simulink model "Modelo_lineal_5GDL_2022"  (R2021b)
settings: Solver=VariableStepAuto  StartTime=0.0  StopTime=0.1  MaxStep=1e-5  RelTol=1e-6
values from neighbouring files (symbols this model uses):
  g = 9.81    [main.m]
undefined symbols (not defined in the file or in its folder): A_EMS, A_HEMS, AG0, B_EMS, B_HEMS, beta, C_EMS, C_HEMS, D_EMS, D_HEMS, dTSensor, filterConstant, I_front, I_rear, initial_conds, noiseSensor, pod, ROTX_0, ROTY_0, ROTZ_0, y_ini, z_0, z_ini
libraries: shared6dof x1
(part 1 of 2)
settings Model: Creator=emate  LastModifiedBy=emate

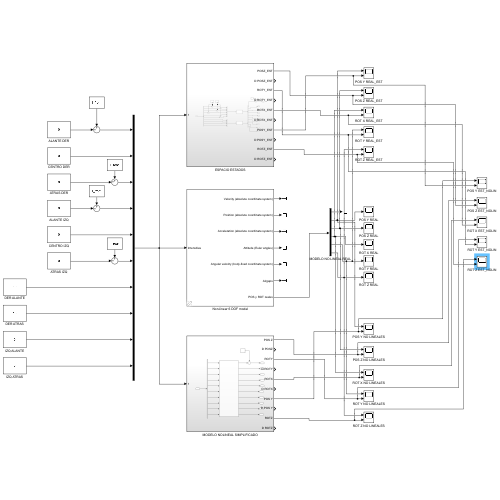
[thumbnail: Simulink's stored preview of the top-level diagram]
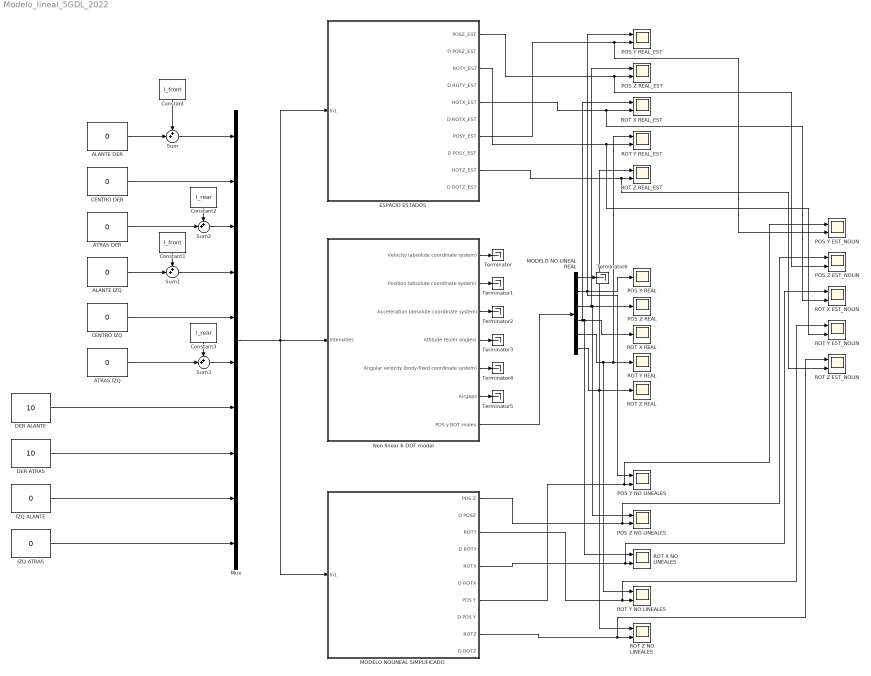
== system Modelo_lineal_5GDL_2022 ==
  ALANTE DER : Constant  Value=0
  ALANTE IZQ : Constant  Value=0
  ATRAS DER : Constant  Value=0
  ATRAS IZQ : Constant  Value=0
  CENTRO DER : Constant  Value=0
  CENTRO IZQ : Constant  Value=0
  Constant : Constant  Value=I_front
  Constant1 : Constant  Value=I_front
  Constant2 : Constant  Value=I_rear
  Constant3 : Constant  Value=I_rear
  DER ALANTE : Constant  Value=10
  DER ATRAS : Constant  Value=10
  ESPACIO ESTADOS : Subsystem
  IZQ ALANTE : Constant  Value=0
  IZQ ATRAS : Constant  Value=0
  MODELO NO LINEAL REAL : Demux  Outputs=6
  MODELO NOLINEAL SIMPLIFICADO : Subsystem
  Mux : Mux  Inputs=10
  Non-linear 6 DOF model : Subsystem  AncestorBlock=libH7_6DOF/Non-linear 6 DOF model
  POS Y EST_NOLIN : Scope  NumInputPorts=2
  POS Y NO LINEALES : Scope  NumInputPorts=2
  POS Y REAL : Scope
  POS Y REAL_EST : Scope  NumInputPorts=2
  POS Z EST_NOLIN : Scope  NumInputPorts=2
  POS Z NO LINEALES : Scope  NumInputPorts=2
  POS Z REAL : Scope
  POS Z REAL_EST : Scope  NumInputPorts=2
  ROT X EST_NOLIN : Scope  NumInputPorts=2
  ROT X NO LINEALES : Scope  NumInputPorts=2
  ROT X REAL : Scope
  ROT X REAL_EST : Scope  NumInputPorts=2
  ROT Y EST_NOLIN : Scope  NumInputPorts=2
  ROT Y NO LINEALES : Scope  NumInputPorts=2
  ROT Y REAL : Scope
  ROT Y REAL_EST : Scope  NumInputPorts=2
  ROT Z EST_NOLIN : Scope  NumInputPorts=2
  ROT Z NO LINEALES : Scope  NumInputPorts=2
  ROT Z REAL : Scope
  ROT Z REAL_EST : Scope  NumInputPorts=2
  Sum{,1..3} (4 alike) : Sum  Inputs=++|
  Terminator{,1..6} (7 alike) : Terminator
  wires:
  CENTRO DER/1 -> Mux/2
  CENTRO IZQ/1 -> Mux/5
  DER ALANTE/1 -> Mux/7
  DER ATRAS/1 -> Mux/8
  IZQ ALANTE/1 -> Mux/9
  IZQ ATRAS/1 -> Mux/10
  Mux/1 -> ESPACIO ESTADOS/1(In1), MODELO NOLINEAL SIMPLIFICADO/1(In1), Non-linear 6 DOF model/1(Intensities)
  Non-linear 6 DOF model/1(Velocity (absolute coordinate system)) -> Terminator/1
  Non-linear 6 DOF model/2(Position (absolute coordinate system)) -> Terminator1/1
  Non-linear 6 DOF model/3(Acceleration (absolute coordinate system)) -> Terminator2/1
  Non-linear 6 DOF model/4(Attitude (Euler angles)) -> Terminator3/1
  Non-linear 6 DOF model/5(Angular velocity (body-fixed coordinate system)) -> Terminator4/1
  Non-linear 6 DOF model/6(Airgaps) -> Terminator5/1
  Non-linear 6 DOF model/7(POS y ROT reales) -> MODELO NO LINEAL REAL/1
  MODELO NO LINEAL REAL/2 -> POS Y NO LINEALES/1, POS Y REAL_EST/1, POS Y REAL/1
  MODELO NO LINEAL REAL/1 -> Terminator6/1
  MODELO NO LINEAL REAL/3 -> POS Z REAL_EST/1, POS Z NO LINEALES/1, POS Z REAL/1
  MODELO NO LINEAL REAL/4 -> ROT X REAL/1, ROT X NO LINEALES/1, ROT X REAL_EST/1
  MODELO NO LINEAL REAL/5 -> ROT Y REAL_EST/1, ROT Y REAL/1, ROT Y NO LINEALES/1
  MODELO NO LINEAL REAL/6 -> ROT Z REAL_EST/1, ROT Z REAL/1, ROT Z NO LINEALES/1
  MODELO NOLINEAL SIMPLIFICADO/7(POS Y) -> POS Y EST_NOLIN/1, POS Y NO LINEALES/2
  MODELO NOLINEAL SIMPLIFICADO/1(POS Z) -> POS Z EST_NOLIN/1, POS Z NO LINEALES/2
  MODELO NOLINEAL SIMPLIFICADO/5(ROTX) -> ROT X EST_NOLIN/1, ROT X NO LINEALES/2
  MODELO NOLINEAL SIMPLIFICADO/3(ROTY) -> ROT Y EST_NOLIN/1, ROT Y NO LINEALES/2
  MODELO NOLINEAL SIMPLIFICADO/9(ROTZ) -> ROT Z EST_NOLIN/1, ROT Z NO LINEALES/2
  ESPACIO ESTADOS/7(POSY_EST) -> POS Y EST_NOLIN/2, POS Y REAL_EST/2
  ESPACIO ESTADOS/1(POSZ_EST) -> POS Z EST_NOLIN/2, POS Z REAL_EST/2
  ESPACIO ESTADOS/5(ROTX_EST) -> ROT X REAL_EST/2, ROT X EST_NOLIN/2
  ESPACIO ESTADOS/3(ROTY_EST) -> ROT Y REAL_EST/2, ROT Y EST_NOLIN/2
  ESPACIO ESTADOS/9(ROTZ_EST) -> ROT Z EST_NOLIN/2, ROT Z REAL_EST/2
  Sum/1 -> Mux/1
  ALANTE DER/1 -> Sum/2
  Constant/1 -> Sum/1
  ALANTE IZQ/1 -> Sum1/2
  Sum1/1 -> Mux/4
  Constant1/1 -> Sum1/1
  ATRAS DER/1 -> Sum2/2
  Sum2/1 -> Mux/3
  Constant2/1 -> Sum2/1
  ATRAS IZQ/1 -> Sum3/2
  Sum3/1 -> Mux/6
  Constant3/1 -> Sum3/1

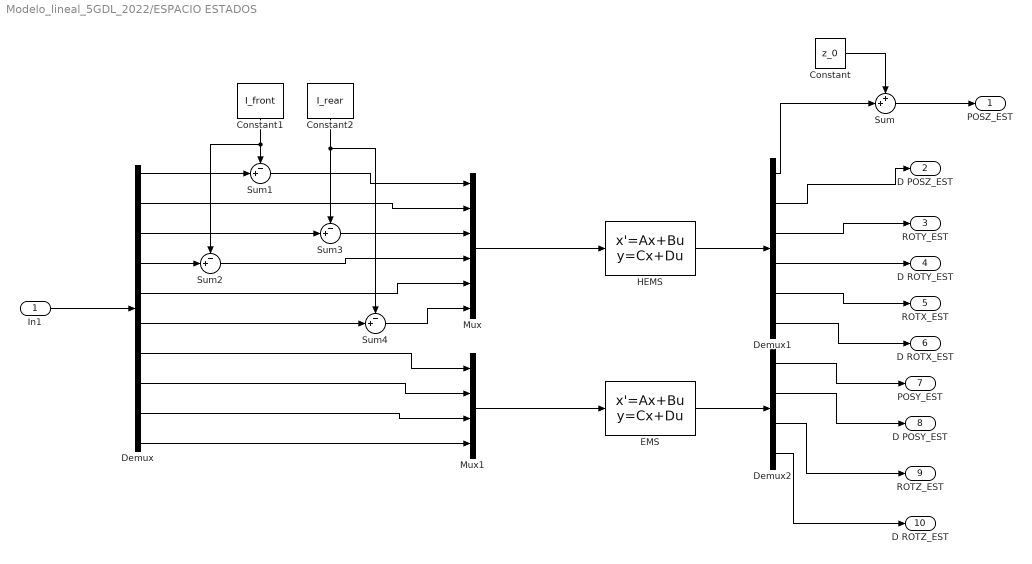
== system Modelo_lineal_5GDL_2022/ESPACIO ESTADOS ==
  In1 : Inport
  Constant : Constant  Value=z_0
  Constant1 : Constant  Value=I_front
  Constant2 : Constant  Value=I_rear
  Demux : Demux  Outputs=10
  Demux1 : Demux  Outputs=6
  Demux2 : Demux
  EMS : StateSpace  A=A_EMS  B=B_EMS  C=C_EMS  D=D_EMS  InitialCondition=[0 0 0 0]
  HEMS : StateSpace  A=A_HEMS  B=B_HEMS  C=C_HEMS  D=D_HEMS  InitialCondition=[0 0 0 0 0 0]
  Mux : Mux  Inputs=6
  Mux1 : Mux
  Sum : Sum  Inputs=++|
  Sum{1..4} (4 alike) : Sum  Inputs=-+|
  POSZ_EST : Outport
  D POSZ_EST : Outport  Port=2
  ROTY_EST : Outport  Port=3
  D ROTY_EST : Outport  Port=4
  ROTX_EST : Outport  Port=5
  D ROTX_EST : Outport  Port=6
  POSY_EST : Outport  Port=7
  D POSY_EST : Outport  Port=8
  ROTZ_EST : Outport  Port=9
  D ROTZ_EST : Outport  Port=10
  wires:
  EMS/1 -> Demux2/1
  HEMS/1 -> Demux1/1
  In1/1 -> Demux/1
  Demux/2 -> Mux/2
  Demux/5 -> Mux/5
  Mux/1 -> HEMS/1
  Mux1/1 -> EMS/1
  Demux/7 -> Mux1/1
  Demux/8 -> Mux1/2
  Demux/9 -> Mux1/3
  Demux/10 -> Mux1/4
  Demux1/1 -> Sum/2
  Demux1/2 -> D POSZ_EST/1
  Demux1/3 -> ROTY_EST/1
  Demux1/4 -> D ROTY_EST/1
  Demux1/5 -> ROTX_EST/1
  Demux1/6 -> D ROTX_EST/1
  Demux2/1 -> POSY_EST/1
  Demux2/2 -> D POSY_EST/1
  Demux2/3 -> ROTZ_EST/1
  Demux2/4 -> D ROTZ_EST/1
  Sum/1 -> POSZ_EST/1
  Constant/1 -> Sum/1
  Demux/1 -> Sum1/2
  Sum1/1 -> Mux/1
  Constant1/1 -> Sum2/1, Sum1/1
  Demux/4 -> Sum2/2
  Sum2/1 -> Mux/4
  Demux/3 -> Sum3/2
  Sum3/1 -> Mux/3
  Constant2/1 -> Sum4/1, Sum3/1
  Demux/6 -> Sum4/2
  Sum4/1 -> Mux/6

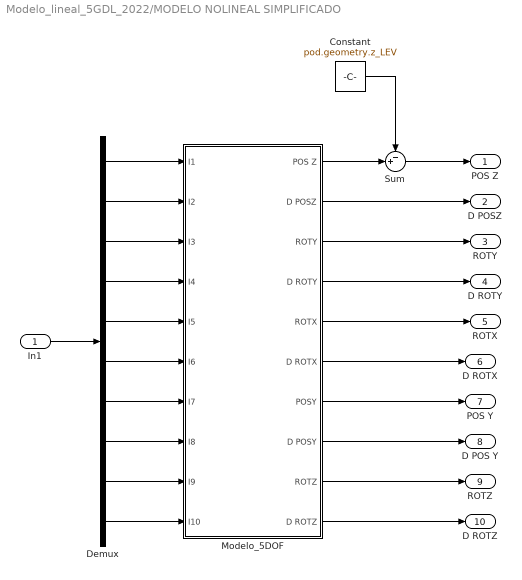
== system Modelo_lineal_5GDL_2022/MODELO NOLINEAL SIMPLIFICADO ==
  In1 : Inport
  Constant : Constant  Value=pod.geometry.z_LEV
  Demux : Demux  Outputs=10
  Modelo_5DOF : Subsystem
  Sum : Sum  Inputs=-+|
  POS Z : Outport
  D POSZ : Outport  Port=2
  ROTY : Outport  Port=3
  D ROTY : Outport  Port=4
  ROTX : Outport  Port=5
  D ROTX : Outport  Port=6
  POS Y : Outport  Port=7
  D POS Y : Outport  Port=8
  ROTZ : Outport  Port=9
  D ROTZ : Outport  Port=10
  wires:
  Demux/7 -> Modelo_5DOF/7(I7)
  Demux/8 -> Modelo_5DOF/8(I8)
  Demux/5 -> Modelo_5DOF/5(I5)
  Demux/2 -> Modelo_5DOF/2(I2)
  Demux/3 -> Modelo_5DOF/3(I3)
  Demux/6 -> Modelo_5DOF/6(I6)
  Demux/1 -> Modelo_5DOF/1(I1)
  Demux/4 -> Modelo_5DOF/4(I4)
  Demux/10 -> Modelo_5DOF/10(I10)
  Demux/9 -> Modelo_5DOF/9(I9)
  In1/1 -> Demux/1
  Modelo_5DOF/1(POS Z) -> Sum/2
  Constant/1 -> Sum/1
  Sum/1 -> POS Z/1
  Modelo_5DOF/2(D POSZ) -> D POSZ/1
  Modelo_5DOF/3(ROTY) -> ROTY/1
  Modelo_5DOF/4(D ROTY) -> D ROTY/1
  Modelo_5DOF/5(ROTX) -> ROTX/1
  Modelo_5DOF/6(D ROTX) -> D ROTX/1
  Modelo_5DOF/7(POSY) -> POS Y/1
  Modelo_5DOF/8(D POSY) -> D POS Y/1
  Modelo_5DOF/9(ROTZ) -> ROTZ/1
  Modelo_5DOF/10(D ROTZ) -> D ROTZ/1

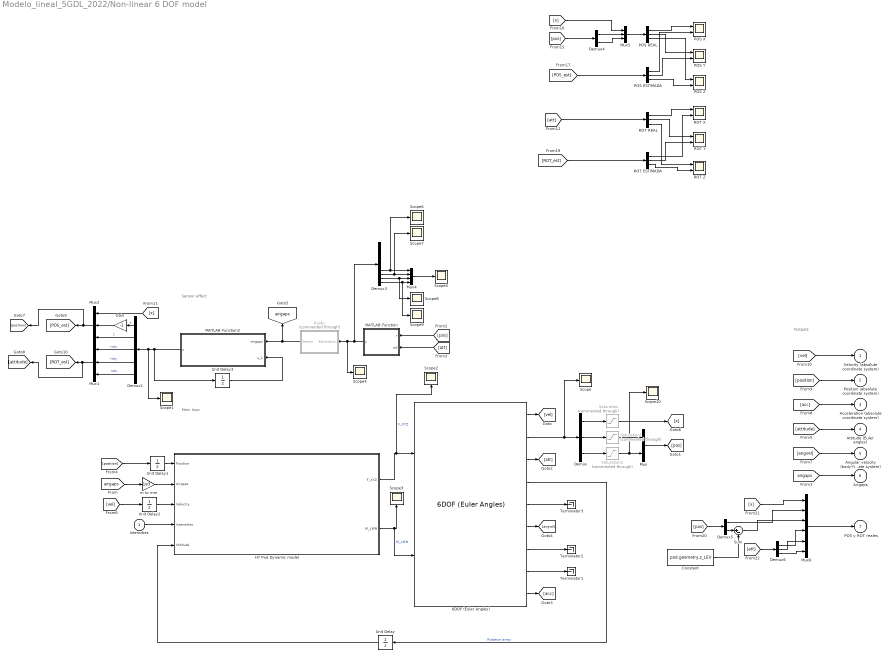
== system Modelo_lineal_5GDL_2022/Non-linear 6 DOF model ==
  note: Sensor effect
  note: Main loop
  note: Outputs
  Intensities : Inport
  " ROT X" : Scope  NumInputPorts=2
  " ROT Y" : Scope  NumInputPorts=2
  " ROT Z" : Scope  NumInputPorts=2
  6DOF (Euler Angles) : shared6dof/6DOF (Euler Angles)  units=Metric (MKS)  mtype=Fixed  rep=Euler Angles  xme_0=initial_conds.x_0  Vm_0=initial_conds.v_0  eul_0=initial_conds.ang_0  pm_0=initial_conds.w_0  mass_0=pod.mass.mass  mass_e=0.5  mass_f=2.0  inertia=pod.mass.inertia  inertia_e=eye(3)  inertia_f=2*eye(3)  k_quat=1.0  vre_flag=on  abi_flag=on  aMode=0  xme_statename=''  Vm_statename=''  eul_statename=''  quat_statename=''  pm_statename=''  mass_statename=''
      link override Abi: Port=9
      settings: SourceProductBaseCode=AE,PW,DR,MT,UV,VE
  Constant : Constant  Value=pod.geometry.z_LEV
  Demux : Demux  Outputs=3
  Demux1 : Demux  Outputs=5
  Demux3 : Demux  Outputs=10
  Demux4 : Demux  Outputs=2
  Demux5 : Demux  Outputs=2
  Demux6 : Demux  Outputs=3
  Gain : Gain  Gain=-1
  H7 Pod Dynamic model : Subsystem  AncestorBlock=libH7_6DOF/H7 Pod Dynamic model
      mask Display: image('FBD.png', [0.12 0.12 0.78 0.78]); % Use "Edit Image" on toolstrip to change.
  MATLAB Function : MATLAB Function  TreatAsAtomicUnit=on
  MATLAB Function2 : MATLAB Function  TreatAsAtomicUnit=on
  Mux : Mux  Inputs=2
  Mux1 : Mux  Inputs=3
  Mux2 : Mux  Inputs=3
  Mux4 : Mux
  Mux5 : Mux  Inputs=3
  Mux6 : Mux  Inputs=6
  POS ESTIMADA : Demux  Outputs=3
  POS REAL : Demux  Outputs=3
  POS X : Scope  NumInputPorts=2
  POS Y : Scope  NumInputPorts=2
  POS Z : Scope  NumInputPorts=2
  ROT ESTIMADA : Demux  Outputs=3
  ROT REAL : Demux  Outputs=3
  Ruido : Subsystem  Commented=through
  Saturation : Saturate  Commented=through  UpperLimit=20  LowerLimit=0
  Saturation1 : Saturate  Commented=through  UpperLimit=0.002  LowerLimit=-0.002
  Saturation2 : Saturate  Commented=through  UpperLimit=0.3504  LowerLimit=0.3384
  Scope{,1..10} (11 alike) : Scope
  Sum : Sum  Inputs=|+-
  Terminator1 : Terminator
  Terminator2 : Terminator
  Terminator3 : Terminator
  Unit Delay : UnitDelay  InitialCondition=eye(3,3)  SampleTime=-1  HasFrameUpgradeWarning=on
  Unit Delay1 : UnitDelay  InitialCondition=initial_conds.x_0  SampleTime=-1  HasFrameUpgradeWarning=on
  Unit Delay2 : UnitDelay  InitialCondition=initial_conds.v_0  SampleTime=-1  HasFrameUpgradeWarning=on
  Unit Delay3 : UnitDelay  SampleTime=-1  HasFrameUpgradeWarning=on
  m to mm : Gain  Gain=1e3
  Velocity (absolute coordinate system) : Outport
  Position (absolute coordinate system) : Outport  Port=2
  Acceleration (absolute coordinate system) : Outport  Port=3
  Attitude (Euler angles) : Outport  Port=4
  Angular velocity (body-fixed coordinate system) : Outport  Port=5
  Airgaps : Outport  Port=6
  POS y ROT reales : Outport  Port=7
  tag scope: airgaps=global
  wires:
  Demux1/3 -> Mux1/1  "rotx"
  6DOF (Euler Angles)/8 -> Terminator1/1
  6DOF (Euler Angles)/4 -> Unit Delay/1  "Rotation array"
  6DOF (Euler Angles)/7 -> Terminator2/1
  Unit Delay2/1 -> H7 Pod Dynamic model/3(Velocity)
  Demux/3 -> Saturation2/1
  H7 Pod Dynamic model/2(M_LMN) -> Scope3/1, 6DOF (Euler Angles)/2  "M_LMN"
  H7 Pod Dynamic model/1(F_XYZ) -> Scope2/1, 6DOF (Euler Angles)/1  "F_XYZ"
  Unit Delay/1 -> H7 Pod Dynamic model/5(Attitude)
  6DOF (Euler Angles)/3 -> [att]
  [airgaps] -> m to mm/1
  [position] -> Position (absolute coordinate system)/1
  [vel] -> Velocity (absolute coordinate system)/1
  [airgaps] -> Airgaps/1
  Unit Delay1/1 -> H7 Pod Dynamic model/1(Position)
  [angvel] -> Angular velocity (body-fixed coordinate system)/1
  6DOF (Euler Angles)/6 -> [angvel]
  6DOF (Euler Angles)/2 -> Scope/1, Demux/1
  Demux/2 -> Saturation1/1
  6DOF (Euler Angles)/9 -> [acc]
  [pos] -> MATLAB Function/1(r)
  MATLAB Function2/1(u) -> Unit Delay3/1, Scope1/1, Demux1/1
  [attitude] -> Attitude (Euler angles)/1
  Mux/1 -> [pos]
  Saturation/1 -> [x]
  [att] -> MATLAB Function/2(rot)
  Demux1/2 -> Mux2/3  "z"
  MATLAB Function/1(y) -> Demux3/1, Ruido/1(Estimation), Scope4/1
  Intensities/1 -> H7 Pod Dynamic model/4(Intensities)
  [position] -> Unit Delay1/1
  Unit Delay3/1 -> MATLAB Function2/2(u_1)
  6DOF (Euler Angles)/1 -> [vel]
  Demux1/4 -> Mux1/2  "roty"
  Demux1/5 -> Mux1/3  "rotz"
  [vel] -> Unit Delay2/1
  Demux/1 -> Saturation/1
  Ruido/1(Sensor) -> [airgaps], MATLAB Function2/1(airgaps)
  [x] -> Mux2/1
  Saturation1/1 -> Mux/1
  Demux1/1 -> Gain/1  "y"
  6DOF (Euler Angles)/5 -> Terminator3/1
  [acc] -> Acceleration (absolute coordinate system)/1
  Saturation2/1 -> Scope10/1, Mux/2
  m to mm/1 -> H7 Pod Dynamic model/2(Airgaps)
  Demux3/7 -> Scope6/1, Mux4/1
  Demux3/8 -> Scope7/1, Mux4/2
  Demux3/9 -> Scope8/1, Mux4/3
  Demux3/10 -> Scope9/1, Mux4/4
  Mux4/1 -> Scope5/1
  Mux2/1 -> [position], [POS_est]
  Mux1/1 -> [attitude], [ROT_est]
  [pos] -> Demux4/1
  [x] -> Mux5/1
  Demux4/1 -> Mux5/2
  Demux4/2 -> Mux5/3
  Mux5/1 -> POS REAL/1
  [POS_est] -> POS ESTIMADA/1
  POS REAL/1 -> POS X/1
  POS ESTIMADA/1 -> POS X/2
  POS REAL/2 -> POS Y/1
  POS ESTIMADA/2 -> POS Y/2
  POS ESTIMADA/3 -> POS Z/2
  POS REAL/3 -> POS Z/1
  [att] -> ROT REAL/1
  [ROT_est] -> ROT ESTIMADA/1
  ROT REAL/1 -> " ROT X"/1
  ROT ESTIMADA/1 -> " ROT X"/2
  ROT REAL/2 -> " ROT Y"/1
  ROT ESTIMADA/2 -> " ROT Y"/2
  ROT REAL/3 -> " ROT Z"/1
  ROT ESTIMADA/3 -> " ROT Z"/2
  Gain/1 -> Mux2/2
  [pos] -> Demux5/1
  [att] -> Demux6/1
  Mux6/1 -> POS y ROT reales/1
  [x] -> Mux6/1
  Demux5/1 -> Mux6/2
  Demux6/1 -> Mux6/4
  Demux6/2 -> Mux6/5
  Demux6/3 -> Mux6/6
  Demux5/2 -> Sum/1
  Sum/1 -> Mux6/3
  Constant/1 -> Sum/2

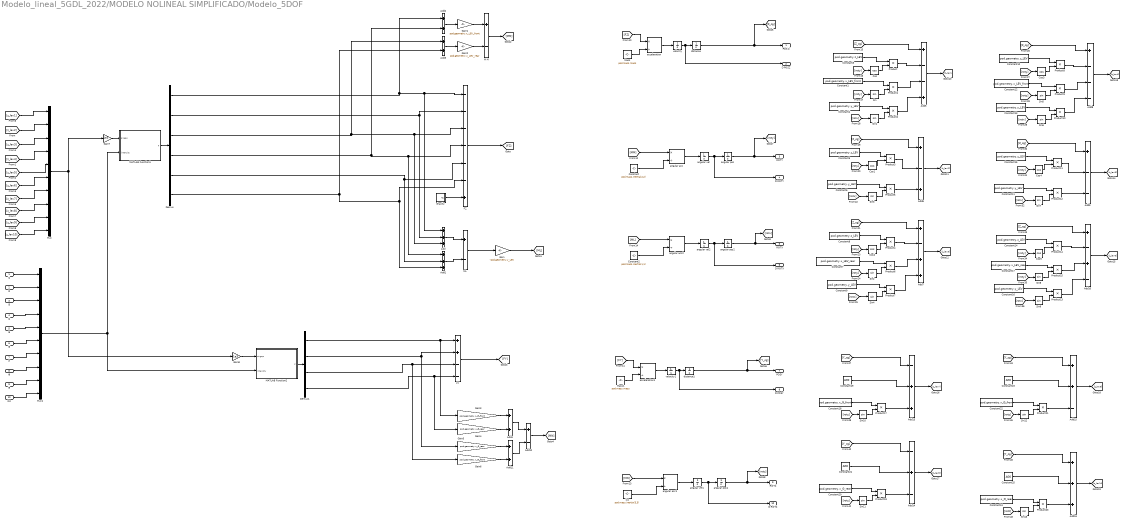
== system Modelo_lineal_5GDL_2022/MODELO NOLINEAL SIMPLIFICADO/Modelo_5DOF ==
  I1 : Inport
  I2 : Inport  Port=2
  I3 : Inport  Port=3
  I4 : Inport  Port=4
  I5 : Inport  Port=5
  I6 : Inport  Port=6
  I7 : Inport  Port=7
  I8 : Inport  Port=8
  I9 : Inport  Port=9
  I10 : Inport  Port=10
  Add : Sum  Inputs=+++
  Add1 : Sum  Inputs=+++
  Add10 : Sum  Inputs=+-+-
  Add{2..4,11} (4 alike) : Sum
  Add12 : Sum  Inputs=+-
  Add13 : Sum  Inputs=-++
  Add14 : Sum  Inputs=-+-
  Add15 : Sum  Inputs=++-
  Add16 : Sum  Inputs=+++
  Add5 : Sum  Inputs=+--+
  Add6 : Sum  Inputs=+-+
  Add7 : Sum  Inputs=+-++
  Add8 : Sum  Inputs=+---
  Add9 : Sum  Inputs=+--
  Constant : Constant  Value=pod.mass.inertia(2,2)
  Constant1 : Constant  Value=pod.geometry.x_LEV_front
  Constant{3,5,8,10,14..15} (6 alike) : Constant  Value=pod.geometry.z_LEV
  Constant{4,6,9,11,13,16} (6 alike) : Constant  Value=pod.geometry.y_LEV
  Constant12 : Constant  Value=pod.geometry.x_LEV_front
  Constant17 : Constant  Value=pod.geometry.x_LEV_rear
  Constant18 : Constant  Value=pod.geometry.x_G_front
  Constant{19,21,23,25} (4 alike) : Constant  Value=AG0
  Constant2 : Constant  Value=pod.mass.inertia(1,1)
  Constant20 : Constant  Value=pod.geometry.x_G_rear
  Constant22 : Constant  Value=pod.geometry.x_G_front
  Constant24 : Constant  Value=pod.geometry.x_G_rear
  Constant7 : Constant  Value=pod.geometry.x_LEV_rear
  Cos{,1..5} (6 alike) : Trigonometry  Operator=cos
  Demux : Demux  Outputs=6
  Demux1 : Demux
  FY : Sum  Inputs=++--
  FZ : Sum  Inputs=------+
  Gain : Gain  Gain=-pod.geometry.y_LEV
  Gain1 : Gain  Gain=pod.geometry.x_LEV_front
  Gain2 : Gain  Gain=pod.geometry.x_LEV_rear
  Gain3 : Gain  Gain=pod.geometry.x_G_front
  Gain4 : Gain  Gain=pod.geometry.x_G_rear
  Gain5 : Gain  Gain=pod.geometry.x_G_rear
  Gain6 : Gain  Gain=pod.geometry.x_G_front
  Gain7 : Gain  Gain=1e3
  Gain8 : Gain  Gain=1e3
  Gravity : Subsystem
  Izz : Constant  Value=pod.mass.inertia(3,3)
  M M : Sum  Inputs=+-
  MATLAB Function1 : MATLAB Function  TreatAsAtomicUnit=on
  MATLAB Function2 : MATLAB Function  TreatAsAtomicUnit=on
  ML : Sum  Inputs=+-
  Mass : Constant  Value=pod.mass.mass
  Mass1 : Constant  Value=pod.mass.mass
  Mux : Mux  Inputs=10
  Mux1 : Mux  Inputs=10
  Product{,1..15,17,19,21,23} (20 alike) : Product
  Sin{,1..13} (14 alike) : Trigonometry
  acceleration : Product  Inputs=*/
  acceleration1 : Product  Inputs=*/
  angular acc : Product  Inputs=*/
  angular acc1 : Product  Inputs=*/
  angular acc2 : Product  Inputs=*/
  angular pos : Integrator  InitialCondition=ROTY_0
  angular pos1 : Integrator  InitialCondition=ROTZ_0
  angular pos2 : Integrator  InitialCondition=ROTX_0
  angular vel : Integrator
  angular vel1 : Integrator
  angular vel2 : Integrator
  distance : Integrator  InitialCondition=z_ini
  distance1 : Integrator  InitialCondition=y_ini
  velocity : Integrator
  velocity1 : Integrator
  POS Z : Outport  VectorParamsAs1DForOutWhenUnconnected=off
  D POSZ : Outport  Port=2  VectorParamsAs1DForOutWhenUnconnected=off
  ROTY : Outport  Port=3  VectorParamsAs1DForOutWhenUnconnected=off
  D ROTY : Outport  Port=4  VectorParamsAs1DForOutWhenUnconnected=off
  ROTX : Outport  Port=5  VectorParamsAs1DForOutWhenUnconnected=off
  D ROTX : Outport  Port=6  VectorParamsAs1DForOutWhenUnconnected=off
  POSY : Outport  Port=7  VectorParamsAs1DForOutWhenUnconnected=off
  D POSY : Outport  Port=8  VectorParamsAs1DForOutWhenUnconnected=off
  ROTZ : Outport  Port=9  VectorParamsAs1DForOutWhenUnconnected=off
  D ROTZ : Outport  Port=10  VectorParamsAs1DForOutWhenUnconnected=off
  wires:
  acceleration/1 -> velocity/1
  velocity/1 -> D POSZ/1, distance/1
  distance/1 -> [Z_cg], POS Z/1
  Demux/1 -> Add/1, FZ/1, Add2/1
  Demux/2 -> FZ/2, Add/2
  Demux/3 -> Add/3, FZ/3, Add3/1
  Mass/1 -> acceleration/2
  Demux/4 -> Add1/1, FZ/4, Add2/2
  Demux/5 -> Add1/2, FZ/5
  Demux/6 -> Add1/3, FZ/6, Add3/2
  Gravity/1(Fg) -> FZ/7
  FZ/1 -> [FZ]
  ML/1 -> Gain/1
  Add1/1 -> ML/2
  Add/1 -> ML/1
  M M/1 -> [MM]
  Add2/1 -> Gain1/1
  Add3/1 -> Gain2/1
  Gain/1 -> [ML]
  [FZ] -> acceleration/1
  angular vel/1 -> D ROTY/1, angular pos/1
  angular pos/1 -> [roty], ROTY/1
  angular acc/1 -> angular vel/1
  [MM] -> angular acc/1
  Constant/1 -> angular acc/2
  angular pos2/1 -> [rotx], ROTX/1
  [ML] -> angular acc2/1
  angular vel2/1 -> angular pos2/1, D ROTX/1
  Constant2/1 -> angular acc2/2
  angular acc2/1 -> angular vel2/1
  [Z_cg] -> Add5/1
  Constant3/1 -> Product/1
  Cos/1 -> Product/2
  [roty] -> Cos/1
  Product/1 -> Add5/2
  [roty] -> Sin/1
  Sin/1 -> Product1/2
  Constant1/1 -> Product1/1
  Product1/1 -> Add5/3
  Constant4/1 -> Product2/1
  Sin1/1 -> Product2/2
  [rotx] -> Sin1/1
  Product2/1 -> Add5/4
  Add5/1 -> [z_lev1]
  Add6/1 -> [z_lev2]
  [rotx] -> Sin3/1
  Sin3/1 -> Product5/2
  Constant6/1 -> Product5/1
  Product3/1 -> Add6/2
  [roty] -> Cos1/1
  Cos1/1 -> Product3/2
  Constant5/1 -> Product3/1
  [Z_cg] -> Add6/1
  Product5/1 -> Add6/3
  Add7/1 -> [z_lev3]
  Product7/1 -> Add7/4
  [rotx] -> Sin4/1
  Sin4/1 -> Product7/2
  Constant9/1 -> Product7/1
  Product6/1 -> Add7/3
  Constant7/1 -> Product6/1
  Sin2/1 -> Product6/2
  [roty] -> Sin2/1
  Product4/1 -> Add7/2
  [roty] -> Cos2/1
  Cos2/1 -> Product4/2
  Constant8/1 -> Product4/1
  [Z_cg] -> Add7/1
  [Z_cg] -> Add8/1
  Constant10/1 -> Product8/1
  Cos3/1 -> Product8/2
  [roty] -> Cos3/1
  Product8/1 -> Add8/2
  [roty] -> Sin5/1
  Sin5/1 -> Product9/2
  Constant12/1 -> Product9/1
  Product9/1 -> Add8/3
  Constant13/1 -> Product10/1
  Sin6/1 -> Product10/2
  [rotx] -> Sin6/1
  Product10/1 -> Add8/4
  Add8/1 -> [z_lev4]
  Product12/1 -> Add9/3
  [Z_cg] -> Add9/1
  Constant15/1 -> Product11/1
  Cos4/1 -> Product11/2
  [roty] -> Cos4/1
  Product11/1 -> Add9/2
  Constant11/1 -> Product12/1
  Sin7/1 -> Product12/2
  [rotx] -> Sin7/1
  Add9/1 -> [z_lev5]
  Add10/1 -> [z_lev6]
  Product13/1 -> Add10/4
  [rotx] -> Sin9/1
  Sin9/1 -> Product13/2
  Constant16/1 -> Product13/1
  Product15/1 -> Add10/3
  Constant17/1 -> Product15/1
  Sin8/1 -> Product15/2
  [roty] -> Sin8/1
  Product14/1 -> Add10/2
  [roty] -> Cos5/1
  Cos5/1 -> Product14/2
  Constant14/1 -> Product14/1
  [Z_cg] -> Add10/1
  Gain1/1 -> M M/1
  Gain2/1 -> M M/2
  FY/1 -> [FY]
  Demux1/4 -> Gain4/1, FY/4
  Demux1/2 -> FY/2, Gain5/1
  Demux1/3 -> Gain6/1, FY/3
  Demux1/1 -> Gain3/1, FY/1
  Add11/1 -> Add12/2
  Add12/1 -> [MN]
  Gain6/1 -> Add11/2
  Gain5/1 -> Add11/1
  Gain3/1 -> Add4/1
  Gain4/1 -> Add4/2
  Add4/1 -> Add12/1
  distance1/1 -> [Y_cg], POSY/1
  angular vel1/1 -> D ROTZ/1, angular pos1/1
  Mass1/1 -> acceleration1/2
  [FY] -> acceleration1/1
  angular acc1/1 -> angular vel1/1
  Izz/1 -> angular acc1/2
  velocity1/1 -> distance1/1, D POSY/1
  angular pos1/1 -> [rotz], ROTZ/1
  acceleration1/1 -> velocity1/1
  [MN] -> angular acc1/1
  Sin11/1 -> Product19/2
  Product19/1 -> Add14/3
  [Y_cg] -> Add14/1
  [Y_cg] -> Add13/1
  Constant18/1 -> Product17/1
  Product17/1 -> Add13/3
  Constant19/1 -> Add13/2
  Add13/1 -> [z_lev7]
  [rotz] -> Sin10/1
  Constant20/1 -> Product19/1
  Sin10/1 -> Product17/2
  Constant21/1 -> Add14/2
  [rotz] -> Sin11/1
  Add14/1 -> [z_lev8]
  Constant25/1 -> Add16/2
  Constant23/1 -> Add15/2
  [Y_cg] -> Add15/1
  Constant22/1 -> Product21/1
  [rotz] -> Sin13/1
  [Y_cg] -> Add16/1
  Add16/1 -> [z_lev10]
  Product21/1 -> Add15/3
  Sin13/1 -> Product23/2
  [rotz] -> Sin12/1
  Add15/1 -> [z_lev9]
  Constant24/1 -> Product23/1
  Sin12/1 -> Product21/2
  Product23/1 -> Add16/3
  MATLAB Function1/1(F) -> Demux/1
  Gain7/1 -> MATLAB Function1/1(airgap)
  MATLAB Function2/1(F) -> Demux1/1
  Gain8/1 -> MATLAB Function2/1(airgap)
  [z_lev1] -> Mux/1
  [z_lev2] -> Mux/2
  [z_lev3] -> Mux/3
  [z_lev4] -> Mux/4
  [z_lev5] -> Mux/5
  [z_lev6] -> Mux/6
  [z_lev7] -> Mux/7
  [z_lev8] -> Mux/8
  [z_lev9] -> Mux/9
  [z_lev10] -> Mux/10
  Mux/1 -> Gain8/1, Gain7/1
  I1/1 -> Mux1/1
  I2/1 -> Mux1/2
  I3/1 -> Mux1/3
  I4/1 -> Mux1/4
  I5/1 -> Mux1/5
  I6/1 -> Mux1/6
  I7/1 -> Mux1/7
  I8/1 -> Mux1/8
  I9/1 -> Mux1/9
  I10/1 -> Mux1/10
  Mux1/1 -> MATLAB Function2/2(intensity), MATLAB Function1/2(intensity)

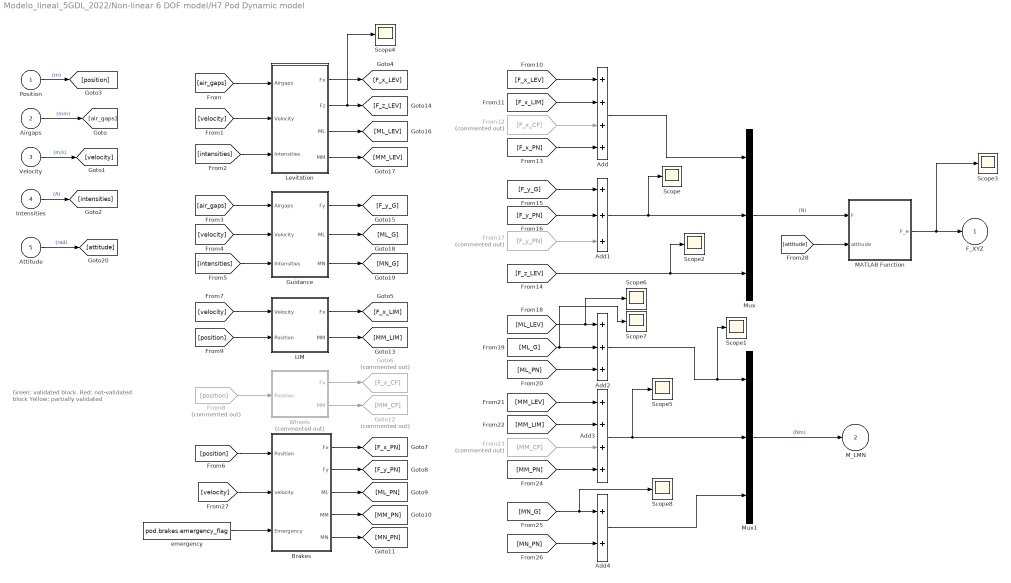
== system Modelo_lineal_5GDL_2022/Non-linear 6 DOF model/H7 Pod Dynamic model ==
  note: Green: validated block.
      | Red: not-validated block
      | Yellow: partially validated
  Position : Inport
  Airgaps : Inport  Port=2
  Velocity : Inport  Port=3
  Intensities : Inport  Port=4
  Attitude : Inport  Port=5
  Add : Sum  Inputs=++++
  Add1 : Sum  Inputs=+++
  Add2 : Sum  Inputs=+++
  Add3 : Sum  Inputs=++++
  Add4 : Sum
  Brakes : Subsystem
  From12 : From  Commented=on  GotoTag=F_x_CF
  From17 : From  Commented=on  GotoTag=F_y_PN
  From23 : From  Commented=on  GotoTag=MM_CF
  From8 : From  Commented=on  GotoTag=position
  Goto12 : Goto  Commented=on  GotoTag=MM_CF
  Goto6 : Goto  Commented=on  GotoTag=F_x_CF
  Guidance : Subsystem
  LIM : Subsystem
  Levitation : Subsystem
  MATLAB Function : MATLAB Function  TreatAsAtomicUnit=on
  Mux : Mux  Inputs=3
  Mux1 : Mux  Inputs=3
  Scope{,1..8} (9 alike) : Scope
  Wheels : Subsystem  Commented=on
  emergency : Constant  Value=pod.brakes.emergency_flag
  F_XYZ : Outport
  M_LMN : Outport  Port=2
  wires:
  Add3/1 -> Scope5/1, Mux1/2
  [MM_LEV] -> Add3/1
  [MM_LIM] -> Add3/2
  [ML_LEV] -> Scope6/1, Add2/1
  Add2/1 -> Scope1/1, Mux1/1
  Add1/1 -> Scope/1, Mux/2
  [F_z_LEV] -> Scope2/1, Mux/3
  From12/1 -> Add/3
  [F_y_PN] -> Add1/2
  MATLAB Function/1(F_e) -> Scope3/1, F_XYZ/1
  Wheels/2(MM) -> Goto12/1
  [air_gaps] -> Levitation/1(Airgaps)
  Brakes/5(MN) -> [MN_PN]
  [F_x_LIM] -> Add/2
  Brakes/4(MM) -> [MM_PN]
  Levitation/2(Fz) -> Scope4/1, [F_z_LEV]
  Guidance/3(MN) -> [MN_G]
  [F_x_LEV] -> Add/1
  Guidance/2(ML) -> [ML_G]
  Attitude/1 -> [attitude]  "(rad)"
  From17/1 -> Add1/3
  emergency/1 -> Brakes/3(Emergency)
  Add/1 -> Mux/1
  Add4/1 -> Mux1/3
  LIM/2(MM) -> [MM_LIM]
  [F_x_PN] -> Add/4
  Brakes/2(Fy) -> [F_y_PN]
  Levitation/4(MM) -> [MM_LEV]
  Wheels/1(Fx) -> Goto6/1
  Levitation/1(Fx) -> [F_x_LEV]
  [MM_PN] -> Add3/4
  Guidance/1(Fy) -> [F_y_G]
  From8/1 -> Wheels/1(Position)
  Brakes/1(Fx) -> [F_x_PN]
  Position/1 -> [position]  "(m)"
  [intensities] -> Levitation/3(Intensities)
  [position] -> Brakes/1(Position)
  [attitude] -> MATLAB Function/2(attitude)
  [position] -> LIM/2(Position)
  [MN_G] -> Scope8/1, Add4/1
  [velocity] -> Brakes/2(velocity)
  [velocity] -> Levitation/2(Velocity)
  [MN_PN] -> Add4/2
  Levitation/3(ML) -> [ML_LEV]
  Brakes/3(ML) -> [ML_PN]
  [velocity] -> LIM/1(Velocity)
  LIM/1(Fx) -> [F_x_LIM]
  [air_gaps] -> Guidance/1(Airgaps)
  [intensities] -> Guidance/3(Intensities)
  Mux1/1 -> M_LMN/1  "(Nm)"
  [F_y_G] -> Add1/1
  From23/1 -> Add3/3
  [velocity] -> Guidance/2(Velocity)
  Mux/1 -> MATLAB Function/1(F)  "(N)"
  [ML_PN] -> Add2/3
  Intensities/1 -> [intensities]  "(A)"
  Velocity/1 -> [velocity]  "(m/s)"
  Airgaps/1 -> [air_gaps]  "(mm)"
  [ML_G] -> Scope7/1, Add2/2

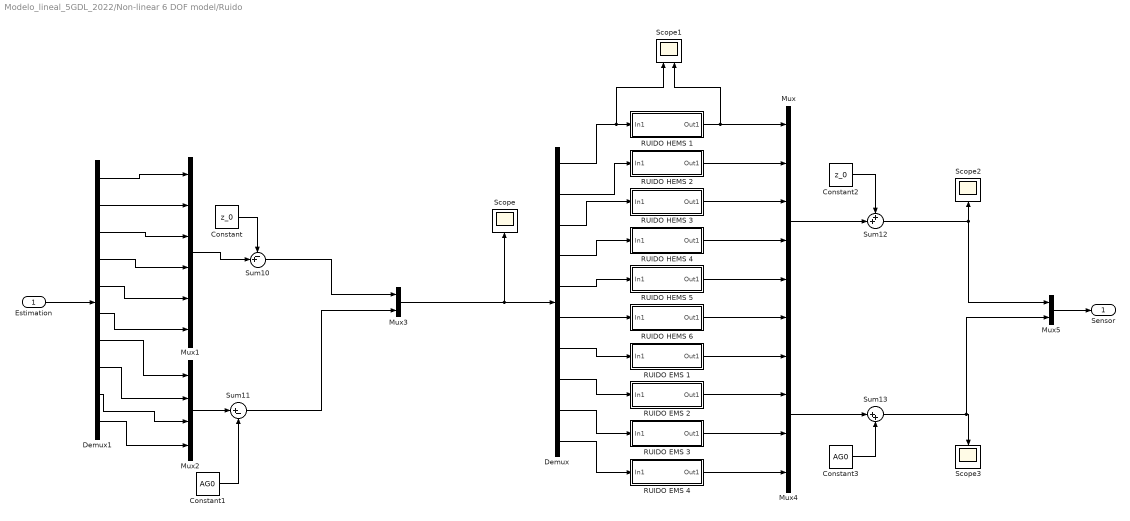
== system Modelo_lineal_5GDL_2022/Non-linear 6 DOF model/Ruido ==
  Estimation : Inport
  Constant : Constant  Value=z_0  SampleTime=dTSensor
  Constant1 : Constant  Value=AG0  SampleTime=dTSensor
  Constant2 : Constant  Value=z_0  SampleTime=dTSensor
  Constant3 : Constant  Value=AG0  SampleTime=dTSensor
  Demux : Demux  Outputs=10
  Demux1 : Demux  Outputs=10
  Mux : Mux  Inputs=6
  Mux1 : Mux  Inputs=6
  Mux2 : Mux
  Mux3 : Mux  Inputs=2
  Mux4 : Mux
  Mux5 : Mux  Inputs=2
  RUIDO EMS 1 : Subsystem
  RUIDO EMS 2 : Subsystem
  RUIDO EMS 3 : Subsystem
  RUIDO EMS 4 : Subsystem
  RUIDO HEMS 1 : Subsystem
  RUIDO HEMS 2 : Subsystem
  RUIDO HEMS 3 : Subsystem
  RUIDO HEMS 4 : Subsystem
  RUIDO HEMS 5 : Subsystem
  RUIDO HEMS 6 : Subsystem
  Scope : Scope
  Scope1 : Scope  NumInputPorts=2
  Scope2 : Scope
  Scope3 : Scope
  Sum10 : Sum  Inputs=-+|
  Sum11 : Sum  Inputs=|+-
  Sum12 : Sum  Inputs=++|
  Sum13 : Sum  Inputs=|++
  Sensor : Outport
  wires:
  Demux1/5 -> Mux1/5
  Mux3/1 -> Demux/1, Scope/1
  Demux1/6 -> Mux1/6
  Sum10/1 -> Mux3/1
  Constant1/1 -> Sum11/2
  Mux2/1 -> Sum11/1
  Demux1/10 -> Mux2/4
  Demux1/2 -> Mux1/2
  Constant/1 -> Sum10/1
  Demux1/7 -> Mux2/1
  Mux1/1 -> Sum10/2
  Demux1/8 -> Mux2/2
  Estimation/1 -> Demux1/1
  Demux1/4 -> Mux1/4
  Demux1/3 -> Mux1/3
  Demux1/1 -> Mux1/1
  Demux1/9 -> Mux2/3
  Sum11/1 -> Mux3/2
  Demux/2 -> RUIDO HEMS 2/1(In1)
  Demux/3 -> RUIDO HEMS 3/1(In1)
  Demux/4 -> RUIDO HEMS 4/1(In1)
  Demux/5 -> RUIDO HEMS 5/1(In1)
  Demux/6 -> RUIDO HEMS 6/1(In1)
  Demux/7 -> RUIDO EMS 1/1(In1)
  Demux/8 -> RUIDO EMS 2/1(In1)
  Demux/9 -> RUIDO EMS 3/1(In1)
  Demux/10 -> RUIDO EMS 4/1(In1)
  RUIDO HEMS 1/1(Out1) -> Scope1/2, Mux/1
  RUIDO HEMS 2/1(Out1) -> Mux/2
  RUIDO HEMS 3/1(Out1) -> Mux/3
  RUIDO HEMS 4/1(Out1) -> Mux/4
  RUIDO HEMS 5/1(Out1) -> Mux/5
  RUIDO HEMS 6/1(Out1) -> Mux/6
  RUIDO EMS 1/1(Out1) -> Mux4/1
  RUIDO EMS 2/1(Out1) -> Mux4/2
  RUIDO EMS 3/1(Out1) -> Mux4/3
  RUIDO EMS 4/1(Out1) -> Mux4/4
  Constant2/1 -> Sum12/1
  Mux/1 -> Sum12/2
  Sum13/1 -> Mux5/2, Scope3/1
  Constant3/1 -> Sum13/2
  Mux4/1 -> Sum13/1
  Sum12/1 -> Mux5/1, Scope2/1
  Mux5/1 -> Sensor/1
  Demux/1 -> Scope1/1, RUIDO HEMS 1/1(In1)

== system Modelo_lineal_5GDL_2022/MODELO NOLINEAL SIMPLIFICADO/Modelo_5DOF/Gravity ==
  Fgrav : Subsystem
  Mass : Constant  Value=pod.mass.mass
  gravity : Constant  Value=g
  Fg : Outport
  wires:
  Fgrav/1(Fg) -> Fg/1
  gravity/1 -> Fgrav/1(gravity)
  Mass/1 -> Fgrav/2(mass)

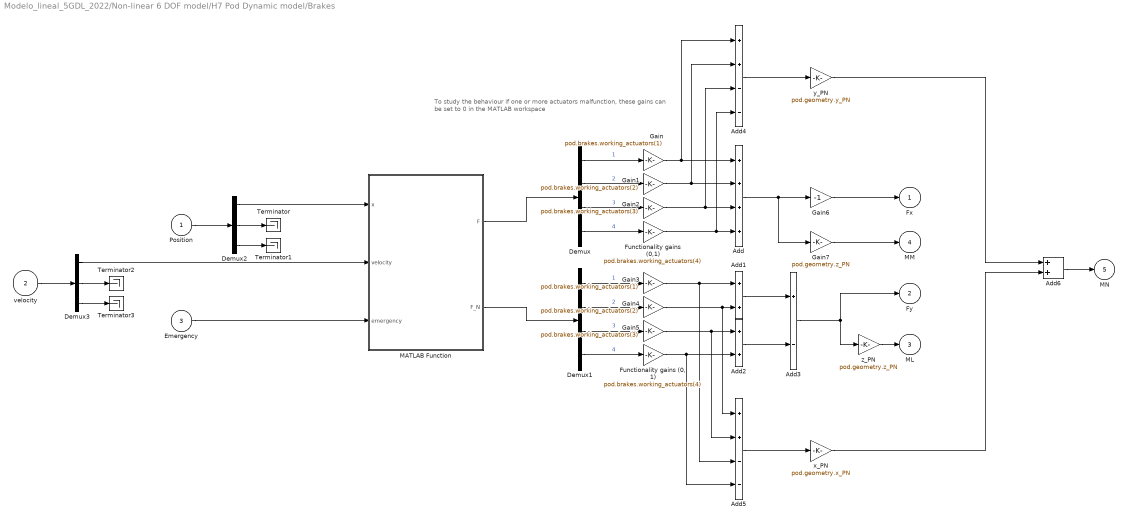
== system Modelo_lineal_5GDL_2022/Non-linear 6 DOF model/H7 Pod Dynamic model/Brakes ==
  note: To study the behaviour if one or more actuators malfunction,
      | these gains can be set to 0 in the MATLAB workspace
  Position : Inport
  velocity : Inport  Port=2
  Emergency : Inport  Port=3
  Add : Sum  Inputs=++++
  Add1 : Sum
  Add2 : Sum
  Add3 : Sum  Inputs=+-
  Add4 : Sum  Inputs=++--
  Add5 : Sum  Inputs=++--
  Add6 : Sum
  Demux : Demux
  Demux1 : Demux
  Demux2 : Demux  Outputs=3
  Demux3 : Demux  Outputs=3
  "Functionality gains (0, 1)" : Gain  Gain=pod.brakes.working_actuators(4)
  Functionality gains (0,1) : Gain  Gain=pod.brakes.working_actuators(4)
  Gain : Gain  Gain=pod.brakes.working_actuators(1)
  Gain1 : Gain  Gain=pod.brakes.working_actuators(2)
  Gain2 : Gain  Gain=pod.brakes.working_actuators(3)
  Gain3 : Gain  Gain=pod.brakes.working_actuators(1)
  Gain4 : Gain  Gain=pod.brakes.working_actuators(2)
  Gain5 : Gain  Gain=pod.brakes.working_actuators(3)
  Gain6 : Gain  Gain=-1
  Gain7 : Gain  Gain=pod.geometry.z_PN
  MATLAB Function : MATLAB Function  TreatAsAtomicUnit=on
  Terminator{,1..3} (4 alike) : Terminator
  x_PN : Gain  Gain=pod.geometry.x_PN
  y_PN : Gain  Gain=pod.geometry.y_PN
  z_PN : Gain  Gain=pod.geometry.z_PN
  Fx : Outport
  Fy : Outport  Port=2
  ML : Outport  Port=3
  MM : Outport  Port=4
  MN : Outport  Port=5
  wires:
  Emergency/1 -> MATLAB Function/3(emergency)
  MATLAB Function/1(F) -> Demux/1
  Demux/1 -> Gain/1  "1"
  Demux/2 -> Gain1/1  "2"
  Demux/3 -> Gain2/1  "3"
  Demux/4 -> Functionality gains (0,1)/1  "4"
  Demux1/4 -> "Functionality gains (0, 1)"/1  "4"
  Demux1/3 -> Gain5/1  "3"
  Demux1/1 -> Gain3/1  "1"
  Demux1/2 -> Gain4/1  "2"
  MATLAB Function/2(F_N) -> Demux1/1
  Functionality gains (0,1)/1 -> Add4/4, Add/4
  Gain2/1 -> Add4/3, Add/3
  Gain1/1 -> Add4/2, Add/2
  Gain/1 -> Add4/1, Add/1
  Add/1 -> Gain7/1, Gain6/1
  Gain6/1 -> Fx/1
  Gain4/1 -> Add5/1, Add1/2
  Gain3/1 -> Add1/1, Add5/3
  Gain5/1 -> Add5/2, Add2/1
  "Functionality gains (0, 1)"/1 -> Add2/2, Add5/4
  Add1/1 -> Add3/1
  Add2/1 -> Add3/2
  Add3/1 -> z_PN/1, Fy/1
  z_PN/1 -> ML/1
  Gain7/1 -> MM/1
  Add4/1 -> y_PN/1
  Demux2/3 -> Terminator1/1
  Position/1 -> Demux2/1
  Demux2/1 -> MATLAB Function/1(x)
  Demux2/2 -> Terminator/1
  velocity/1 -> Demux3/1
  Demux3/2 -> Terminator2/1
  Demux3/3 -> Terminator3/1
  Demux3/1 -> MATLAB Function/2(velocity)
  Add5/1 -> x_PN/1
  Add6/1 -> MN/1
  y_PN/1 -> Add6/1
  x_PN/1 -> Add6/2

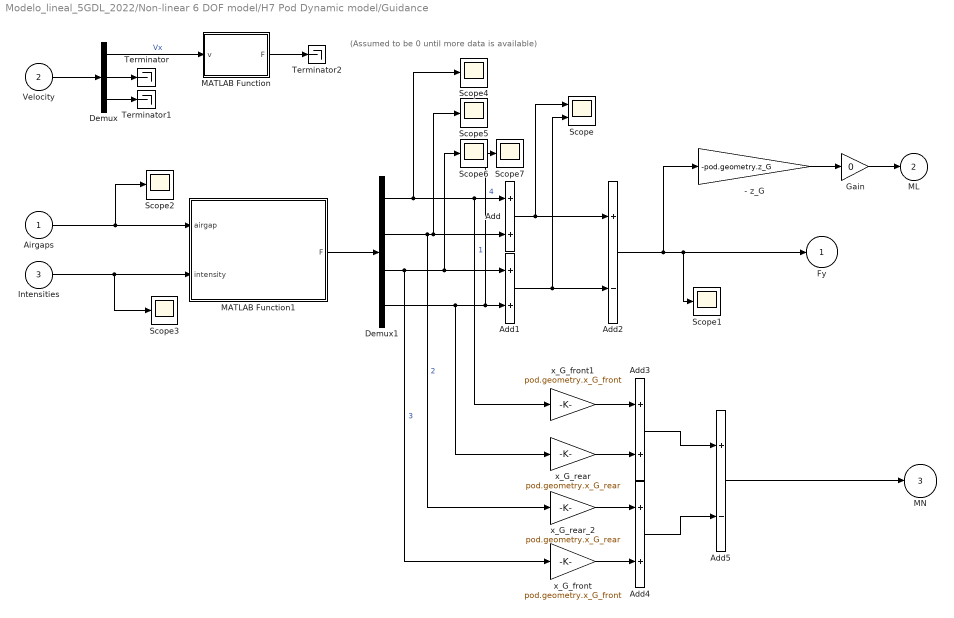
== system Modelo_lineal_5GDL_2022/Non-linear 6 DOF model/H7 Pod Dynamic model/Guidance ==
  note: (Assumed to be 0 until more data is available)
  Airgaps : Inport
  Velocity : Inport  Port=2
  Intensities : Inport  Port=3
  " x_G_front" : Gain  Gain=pod.geometry.x_G_front
  " x_G_front1" : Gain  Gain=pod.geometry.x_G_front
  " x_G_rear" : Gain  Gain=pod.geometry.x_G_rear
  " x_G_rear_2" : Gain  Gain=pod.geometry.x_G_rear
  - z_G : Gain  Gain=-pod.geometry.z_G
  Add{,1,3..4} (4 alike) : Sum
  Add2 : Sum  Inputs=+-
  Add5 : Sum  Inputs=+-
  Demux : Demux  Outputs=3
  Demux1 : Demux
  Gain : Gain  Gain=0
  MATLAB Function : MATLAB Function  TreatAsAtomicUnit=on
  MATLAB Function1 : MATLAB Function  TreatAsAtomicUnit=on
  Scope : Scope  NumInputPorts=2
  Scope{1..7} (7 alike) : Scope
  Terminator : Terminator
  Terminator1 : Terminator
  Terminator2 : Terminator
  Fy : Outport
  ML : Outport  Port=2
  MN : Outport  Port=3
  wires:
  Demux/1 -> MATLAB Function/1(v)  "Vx"
  Velocity/1 -> Demux/1
  Demux/2 -> Terminator/1
  Demux/3 -> Terminator1/1
  MATLAB Function/1(F) -> Terminator2/1
  Intensities/1 -> Scope3/1, MATLAB Function1/2(intensity)
  Airgaps/1 -> Scope2/1, MATLAB Function1/1(airgap)
  Demux1/1 -> Scope4/1, " x_G_front1"/1, Add/1  "1"
  Demux1/2 -> " x_G_rear_2"/1, Scope5/1, Add/2  "2"
  Demux1/3 -> " x_G_front"/1, Scope6/1, Add1/1  "3"
  Demux1/4 -> " x_G_rear"/1, Scope7/1, Add1/2  "4"
  Add1/1 -> Scope/2, Add2/2
  Add/1 -> Scope/1, Add2/1
  Add2/1 -> - z_G/1, Scope1/1, Fy/1
  - z_G/1 -> Gain/1
  Add3/1 -> Add5/1
  Add4/1 -> Add5/2
  Add5/1 -> MN/1
  MATLAB Function1/1(F) -> Demux1/1
  " x_G_front"/1 -> Add4/2
  " x_G_front1"/1 -> Add3/1
  " x_G_rear"/1 -> Add3/2
  " x_G_rear_2"/1 -> Add4/1
  Gain/1 -> ML/1

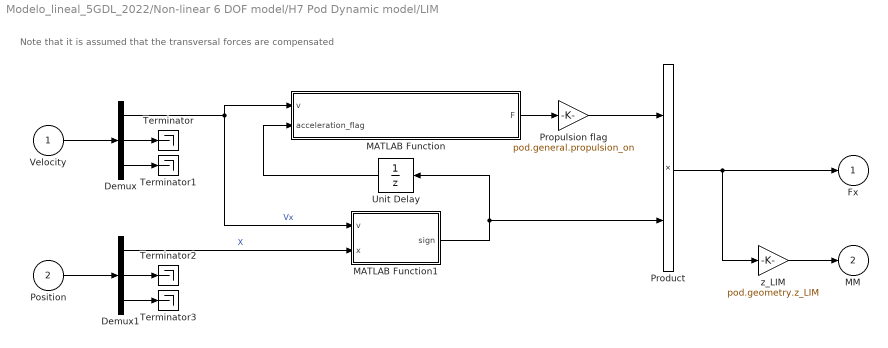
== system Modelo_lineal_5GDL_2022/Non-linear 6 DOF model/H7 Pod Dynamic model/LIM ==
  note: Note that it is assumed that the transversal forces are compensated
  Velocity : Inport
  Position : Inport  Port=2
  Demux : Demux  Outputs=3
  Demux1 : Demux  Outputs=3
  MATLAB Function : MATLAB Function  TreatAsAtomicUnit=on
  MATLAB Function1 : MATLAB Function  TreatAsAtomicUnit=on
  Product : Product
  Propulsion flag : Gain  Gain=pod.general.propulsion_on
  Terminator{,1..3} (4 alike) : Terminator
  Unit Delay : UnitDelay  InitialCondition=1  SampleTime=-1  HasFrameUpgradeWarning=on
  z_LIM : Gain  Gain=pod.geometry.z_LIM
  Fx : Outport
  MM : Outport  Port=2
  wires:
  Unit Delay/1 -> MATLAB Function/2(acceleration_flag)
  Propulsion flag/1 -> Product/1
  Velocity/1 -> Demux/1
  Demux/2 -> Terminator/1
  Demux/3 -> Terminator1/1
  Demux/1 -> MATLAB Function1/1(v), MATLAB Function/1(v)  "Vx"
  Position/1 -> Demux1/1
  Demux1/3 -> Terminator3/1
  Demux1/2 -> Terminator2/1
  Demux1/1 -> MATLAB Function1/2(x)  "X"
  MATLAB Function1/1(sign) -> Product/2, Unit Delay/1
  MATLAB Function/1(F) -> Propulsion flag/1
  Product/1 -> z_LIM/1, Fx/1
  z_LIM/1 -> MM/1

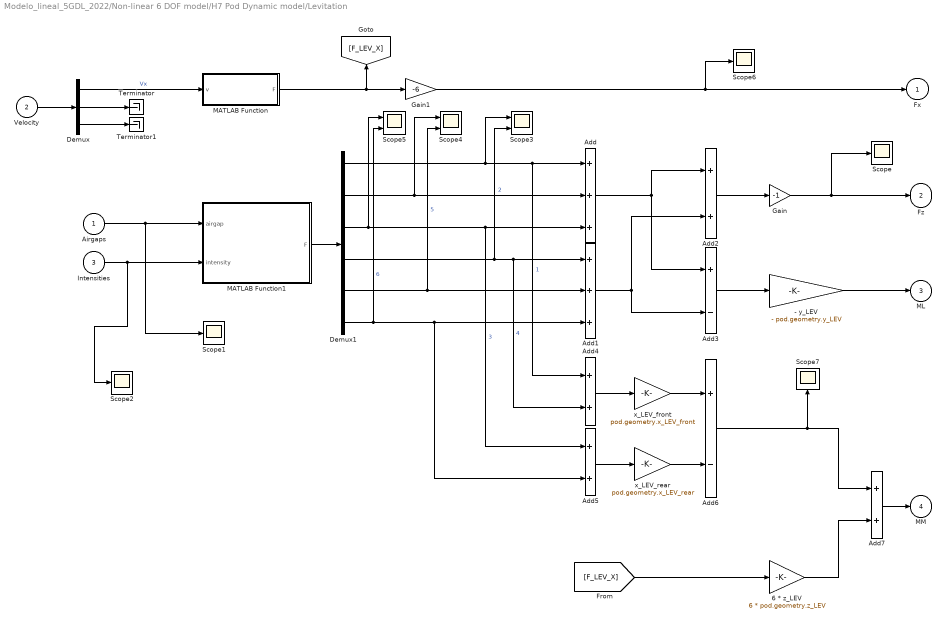
== system Modelo_lineal_5GDL_2022/Non-linear 6 DOF model/H7 Pod Dynamic model/Levitation ==
  Airgaps : Inport
  Velocity : Inport  Port=2
  Intensities : Inport  Port=3
  - y_LEV : Gain  Gain=- pod.geometry.y_LEV
  6 * z_LEV : Gain  Gain=6 * pod.geometry.z_LEV
  Add : Sum  Inputs=+++
  Add1 : Sum  Inputs=+++
  Add{2,4..5,7} (4 alike) : Sum
  Add3 : Sum  Inputs=+-
  Add6 : Sum  Inputs=+-
  Demux : Demux  Outputs=3
  Demux1 : Demux  Outputs=6
  Gain : Gain  Gain=-1
  Gain1 : Gain  Gain=-6
  MATLAB Function : MATLAB Function  TreatAsAtomicUnit=on
  MATLAB Function1 : MATLAB Function  TreatAsAtomicUnit=on
  Scope{,1..2,6..7} (5 alike) : Scope
  Scope3 : Scope  NumInputPorts=2
  Scope4 : Scope  NumInputPorts=2
  Scope5 : Scope  NumInputPorts=2
  Terminator : Terminator
  Terminator1 : Terminator
  x_LEV_front : Gain  Gain=pod.geometry.x_LEV_front
  x_LEV_rear : Gain  Gain=pod.geometry.x_LEV_rear
  Fx : Outport
  Fz : Outport  Port=2
  ML : Outport  Port=3
  MM : Outport  Port=4
  wires:
  Demux/2 -> Terminator/1
  Demux/3 -> Terminator1/1
  Velocity/1 -> Demux/1
  Demux/1 -> MATLAB Function/1(v)  "Vx"
  Airgaps/1 -> MATLAB Function1/1(airgap), Scope1/1
  Intensities/1 -> MATLAB Function1/2(intensity), Scope2/1
  MATLAB Function1/1(F) -> Demux1/1
  Gain/1 -> Fz/1, Scope/1
  Demux1/1 -> Scope3/1, Add4/1, Add/1  "1"
  Demux1/2 -> Scope4/1, Add/2  "2"
  Demux1/3 -> Scope5/1, Add5/1, Add/3  "3"
  Demux1/4 -> Scope3/2, Add4/2, Add1/1  "4"
  Demux1/5 -> Add1/2, Scope4/2  "5"
  Demux1/6 -> Scope5/2, Add5/2, Add1/3  "6"
  Add/1 -> Add2/1, Add3/1
  Add1/1 -> Add2/2, Add3/2
  Add2/1 -> Gain/1
  Add3/1 -> - y_LEV/1
  - y_LEV/1 -> ML/1
  Gain1/1 -> Scope6/1, Fx/1
  [F_LEV_X] -> 6 * z_LEV/1
  Add4/1 -> x_LEV_front/1
  Add5/1 -> x_LEV_rear/1
  Add7/1 -> MM/1
  Add6/1 -> Scope7/1, Add7/1
  6 * z_LEV/1 -> Add7/2
  MATLAB Function/1(F) -> [F_LEV_X], Gain1/1
  x_LEV_front/1 -> Add6/1
  x_LEV_rear/1 -> Add6/2

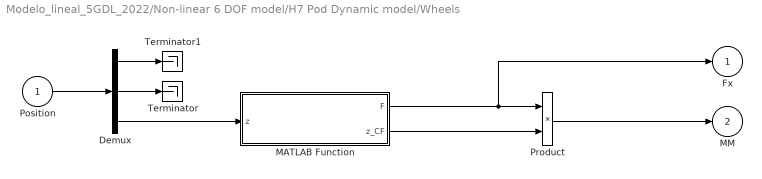
== system Modelo_lineal_5GDL_2022/Non-linear 6 DOF model/H7 Pod Dynamic model/Wheels ==
  Position : Inport
  Demux : Demux  Outputs=3
  MATLAB Function : MATLAB Function  TreatAsAtomicUnit=on
  Product : Product
  Terminator : Terminator
  Terminator1 : Terminator
  Fx : Outport
  MM : Outport  Port=2
  wires:
  Position/1 -> Demux/1
  Demux/2 -> Terminator/1
  Demux/3 -> MATLAB Function/1(z)
  MATLAB Function/1(F) -> Fx/1, Product/1
  Demux/1 -> Terminator1/1
  MATLAB Function/2(z_CF) -> Product/2
  Product/1 -> MM/1

== system Modelo_lineal_5GDL_2022/Non-linear 6 DOF model/Ruido/RUIDO EMS 1 ==
  In1 : Inport
  Filter : Subsystem
  Quantizer : Quantizer  QuantizationInterval=resSensor
  Random Number : RandomNumber  Variance=noiseSensor^2  Seed=24
  Sum : Sum  Inputs=++|
  Zero-Order Hold1 : ZeroOrderHold  SampleTime=dTSensor
  Out1 : Outport
  wires:
  Random Number/1 -> Sum/1
  Zero-Order Hold1/1 -> Filter/1(In1)
  In1/1 -> Sum/2
  Sum/1 -> Quantizer/1
  Quantizer/1 -> Zero-Order Hold1/1
  Filter/1(Out1) -> Out1/1

== system Modelo_lineal_5GDL_2022/Non-linear 6 DOF model/Ruido/RUIDO EMS 2 ==
  In1 : Inport
  Filter : Subsystem
  Quantizer : Quantizer  QuantizationInterval=resSensor
  Random Number : RandomNumber  Variance=noiseSensor^2  Seed=27
  Sum : Sum  Inputs=++|
  Zero-Order Hold1 : ZeroOrderHold  SampleTime=dTSensor
  Out1 : Outport
  wires:
  Filter/1(Out1) -> Out1/1
  Quantizer/1 -> Zero-Order Hold1/1
  Sum/1 -> Quantizer/1
  In1/1 -> Sum/2
  Zero-Order Hold1/1 -> Filter/1(In1)
  Random Number/1 -> Sum/1

== system Modelo_lineal_5GDL_2022/Non-linear 6 DOF model/Ruido/RUIDO EMS 3 ==
  In1 : Inport
  Filter : Subsystem
  Quantizer : Quantizer  QuantizationInterval=resSensor
  Random Number : RandomNumber  Variance=noiseSensor^2  Seed=29
  Sum : Sum  Inputs=++|
  Zero-Order Hold1 : ZeroOrderHold  SampleTime=dTSensor
  Out1 : Outport
  wires:
  Random Number/1 -> Sum/1
  Zero-Order Hold1/1 -> Filter/1(In1)
  In1/1 -> Sum/2
  Sum/1 -> Quantizer/1
  Quantizer/1 -> Zero-Order Hold1/1
  Filter/1(Out1) -> Out1/1

== system Modelo_lineal_5GDL_2022/Non-linear 6 DOF model/Ruido/RUIDO EMS 4 ==
  In1 : Inport
  Filter : Subsystem
  Quantizer : Quantizer  QuantizationInterval=resSensor
  Random Number : RandomNumber  Variance=noiseSensor^2  Seed=30
  Sum : Sum  Inputs=++|
  Zero-Order Hold1 : ZeroOrderHold  SampleTime=dTSensor
  Out1 : Outport
  wires:
  Filter/1(Out1) -> Out1/1
  Quantizer/1 -> Zero-Order Hold1/1
  Sum/1 -> Quantizer/1
  In1/1 -> Sum/2
  Zero-Order Hold1/1 -> Filter/1(In1)
  Random Number/1 -> Sum/1

== system Modelo_lineal_5GDL_2022/Non-linear 6 DOF model/Ruido/RUIDO HEMS 1 ==
  In1 : Inport
  Filter : Subsystem
  Quantizer : Quantizer  QuantizationInterval=resSensor
  Random Number : RandomNumber  Variance=noiseSensor^2  Seed=14
  Sum : Sum  Inputs=++|
  Zero-Order Hold1 : ZeroOrderHold  SampleTime=dTSensor
  Out1 : Outport
  wires:
  Random Number/1 -> Sum/1
  Zero-Order Hold1/1 -> Filter/1(In1)
  In1/1 -> Sum/2
  Sum/1 -> Quantizer/1
  Quantizer/1 -> Zero-Order Hold1/1
  Filter/1(Out1) -> Out1/1

== system Modelo_lineal_5GDL_2022/Non-linear 6 DOF model/Ruido/RUIDO HEMS 2 ==
  In1 : Inport
  Filter : Subsystem
  Quantizer : Quantizer  QuantizationInterval=resSensor
  Random Number : RandomNumber  Variance=noiseSensor^2  Seed=1
  Sum : Sum  Inputs=++|
  Zero-Order Hold1 : ZeroOrderHold  SampleTime=dTSensor
  Out1 : Outport
  wires:
  Filter/1(Out1) -> Out1/1
  Quantizer/1 -> Zero-Order Hold1/1
  Sum/1 -> Quantizer/1
  In1/1 -> Sum/2
  Zero-Order Hold1/1 -> Filter/1(In1)
  Random Number/1 -> Sum/1

== system Modelo_lineal_5GDL_2022/Non-linear 6 DOF model/Ruido/RUIDO HEMS 3 ==
  In1 : Inport
  Filter : Subsystem
  Quantizer : Quantizer  QuantizationInterval=resSensor
  Random Number : RandomNumber  Variance=noiseSensor^2  Seed=3
  Sum : Sum  Inputs=++|
  Zero-Order Hold1 : ZeroOrderHold  SampleTime=dTSensor
  Out1 : Outport
  wires:
  Random Number/1 -> Sum/1
  Zero-Order Hold1/1 -> Filter/1(In1)
  In1/1 -> Sum/2
  Sum/1 -> Quantizer/1
  Quantizer/1 -> Zero-Order Hold1/1
  Filter/1(Out1) -> Out1/1

== system Modelo_lineal_5GDL_2022/Non-linear 6 DOF model/Ruido/RUIDO HEMS 4 ==
  In1 : Inport
  Filter : Subsystem
  Quantizer : Quantizer  QuantizationInterval=resSensor
  Random Number : RandomNumber  Variance=noiseSensor^2  Seed=7
  Sum : Sum  Inputs=++|
  Zero-Order Hold1 : ZeroOrderHold  SampleTime=dTSensor
  Out1 : Outport
  wires:
  Filter/1(Out1) -> Out1/1
  Quantizer/1 -> Zero-Order Hold1/1
  Sum/1 -> Quantizer/1
  In1/1 -> Sum/2
  Zero-Order Hold1/1 -> Filter/1(In1)
  Random Number/1 -> Sum/1

== system Modelo_lineal_5GDL_2022/Non-linear 6 DOF model/Ruido/RUIDO HEMS 5 ==
  In1 : Inport
  Filter : Subsystem
  Quantizer : Quantizer  QuantizationInterval=resSensor
  Random Number : RandomNumber  Variance=noiseSensor^2  Seed=11
  Sum : Sum  Inputs=++|
  Zero-Order Hold1 : ZeroOrderHold  SampleTime=dTSensor
  Out1 : Outport
  wires:
  Random Number/1 -> Sum/1
  Zero-Order Hold1/1 -> Filter/1(In1)
  In1/1 -> Sum/2
  Sum/1 -> Quantizer/1
  Quantizer/1 -> Zero-Order Hold1/1
  Filter/1(Out1) -> Out1/1

== system Modelo_lineal_5GDL_2022/Non-linear 6 DOF model/Ruido/RUIDO HEMS 6 ==
  In1 : Inport
  Filter : Subsystem
  Quantizer : Quantizer  QuantizationInterval=resSensor
  Random Number : RandomNumber  Variance=noiseSensor^2  Seed=21
  Sum : Sum  Inputs=++|
  Zero-Order Hold1 : ZeroOrderHold  SampleTime=dTSensor
  Out1 : Outport
  wires:
  Filter/1(Out1) -> Out1/1
  Quantizer/1 -> Zero-Order Hold1/1
  Sum/1 -> Quantizer/1
  In1/1 -> Sum/2
  Zero-Order Hold1/1 -> Filter/1(In1)
  Random Number/1 -> Sum/1

== system Modelo_lineal_5GDL_2022/MODELO NOLINEAL SIMPLIFICADO/Modelo_5DOF/Gravity/Fgrav ==
  gravity : Inport
  mass : Inport  Port=2
  Product : Product
  Fg : Outport  VectorParamsAs1DForOutWhenUnconnected=off
  wires:
  Product/1 -> Fg/1
  gravity/1 -> Product/1
  mass/1 -> Product/2

== system Modelo_lineal_5GDL_2022/Non-linear 6 DOF model/Ruido/RUIDO EMS 1/Filter ==
  In1 : Inport
  Gain : Gain  Gain=filterConstant
  Gain1 : Gain  Gain=1/(filterConstant+1)
  Sum : Sum  Inputs=|++
  Unit Delay : UnitDelay  SampleTime=dTSensor  HasFrameUpgradeWarning=on
  Out1 : Outport
  wires:
  Gain/1 -> Sum/2
  Sum/1 -> Gain1/1
  Gain1/1 -> Out1/1, Unit Delay/1
  Unit Delay/1 -> Gain/1
  In1/1 -> Sum/1

== system Modelo_lineal_5GDL_2022/Non-linear 6 DOF model/Ruido/RUIDO EMS 2/Filter ==
  In1 : Inport
  Gain : Gain  Gain=filterConstant
  Gain1 : Gain  Gain=1/(filterConstant+1)
  Sum : Sum  Inputs=|++
  Unit Delay : UnitDelay  SampleTime=dTSensor  HasFrameUpgradeWarning=on
  Out1 : Outport
  wires:
  In1/1 -> Sum/1
  Unit Delay/1 -> Gain/1
  Gain1/1 -> Unit Delay/1, Out1/1
  Sum/1 -> Gain1/1
  Gain/1 -> Sum/2

== system Modelo_lineal_5GDL_2022/Non-linear 6 DOF model/Ruido/RUIDO EMS 3/Filter ==
  In1 : Inport
  Gain : Gain  Gain=filterConstant
  Gain1 : Gain  Gain=1/(filterConstant+1)
  Sum : Sum  Inputs=|++
  Unit Delay : UnitDelay  SampleTime=dTSensor  HasFrameUpgradeWarning=on
  Out1 : Outport
  wires:
  Gain/1 -> Sum/2
  Sum/1 -> Gain1/1
  Gain1/1 -> Out1/1, Unit Delay/1
  Unit Delay/1 -> Gain/1
  In1/1 -> Sum/1

== system Modelo_lineal_5GDL_2022/Non-linear 6 DOF model/Ruido/RUIDO EMS 4/Filter ==
  In1 : Inport
  Gain : Gain  Gain=filterConstant
  Gain1 : Gain  Gain=1/(filterConstant+1)
  Sum : Sum  Inputs=|++
  Unit Delay : UnitDelay  SampleTime=dTSensor  HasFrameUpgradeWarning=on
  Out1 : Outport
  wires:
  In1/1 -> Sum/1
  Unit Delay/1 -> Gain/1
  Gain1/1 -> Unit Delay/1, Out1/1
  Sum/1 -> Gain1/1
  Gain/1 -> Sum/2

== system Modelo_lineal_5GDL_2022/Non-linear 6 DOF model/Ruido/RUIDO HEMS 1/Filter ==
  In1 : Inport
  Gain : Gain  Gain=filterConstant
  Gain1 : Gain  Gain=1/(filterConstant+1)
  Sum : Sum  Inputs=|++
  Unit Delay : UnitDelay  SampleTime=dTSensor  HasFrameUpgradeWarning=on
  Out1 : Outport
  wires:
  Gain/1 -> Sum/2
  Sum/1 -> Gain1/1
  Gain1/1 -> Out1/1, Unit Delay/1
  Unit Delay/1 -> Gain/1
  In1/1 -> Sum/1

== system Modelo_lineal_5GDL_2022/Non-linear 6 DOF model/Ruido/RUIDO HEMS 2/Filter ==
  In1 : Inport
  Gain : Gain  Gain=filterConstant
  Gain1 : Gain  Gain=1/(filterConstant+1)
  Sum : Sum  Inputs=|++
  Unit Delay : UnitDelay  SampleTime=dTSensor  HasFrameUpgradeWarning=on
  Out1 : Outport
  wires:
  In1/1 -> Sum/1
  Unit Delay/1 -> Gain/1
  Gain1/1 -> Unit Delay/1, Out1/1
  Sum/1 -> Gain1/1
  Gain/1 -> Sum/2

== system Modelo_lineal_5GDL_2022/Non-linear 6 DOF model/Ruido/RUIDO HEMS 3/Filter ==
  In1 : Inport
  Gain : Gain  Gain=filterConstant
  Gain1 : Gain  Gain=1/(filterConstant+1)
  Sum : Sum  Inputs=|++
  Unit Delay : UnitDelay  SampleTime=dTSensor  HasFrameUpgradeWarning=on
  Out1 : Outport
  wires:
  Gain/1 -> Sum/2
  Sum/1 -> Gain1/1
  Gain1/1 -> Out1/1, Unit Delay/1
  Unit Delay/1 -> Gain/1
  In1/1 -> Sum/1

== system Modelo_lineal_5GDL_2022/Non-linear 6 DOF model/Ruido/RUIDO HEMS 4/Filter ==
  In1 : Inport
  Gain : Gain  Gain=filterConstant
  Gain1 : Gain  Gain=1/(filterConstant+1)
  Sum : Sum  Inputs=|++
  Unit Delay : UnitDelay  SampleTime=dTSensor  HasFrameUpgradeWarning=on
  Out1 : Outport
  wires:
  In1/1 -> Sum/1
  Unit Delay/1 -> Gain/1
  Gain1/1 -> Unit Delay/1, Out1/1
  Sum/1 -> Gain1/1
  Gain/1 -> Sum/2

== system Modelo_lineal_5GDL_2022/Non-linear 6 DOF model/Ruido/RUIDO HEMS 5/Filter ==
  In1 : Inport
  Gain : Gain  Gain=filterConstant
  Gain1 : Gain  Gain=1/(filterConstant+1)
  Sum : Sum  Inputs=|++
  Unit Delay : UnitDelay  SampleTime=dTSensor  HasFrameUpgradeWarning=on
  Out1 : Outport
  wires:
  Gain/1 -> Sum/2
  Sum/1 -> Gain1/1
  Gain1/1 -> Out1/1, Unit Delay/1
  Unit Delay/1 -> Gain/1
  In1/1 -> Sum/1

== system Modelo_lineal_5GDL_2022/Non-linear 6 DOF model/Ruido/RUIDO HEMS 6/Filter ==
  In1 : Inport
  Gain : Gain  Gain=filterConstant
  Gain1 : Gain  Gain=1/(filterConstant+1)
  Sum : Sum  Inputs=|++
  Unit Delay : UnitDelay  SampleTime=dTSensor  HasFrameUpgradeWarning=on
  Out1 : Outport
  wires:
  In1/1 -> Sum/1
  Unit Delay/1 -> Gain/1
  Gain1/1 -> Unit Delay/1, Out1/1
  Sum/1 -> Gain1/1
  Gain/1 -> Sum/2

== matlab function Modelo_lineal_5GDL_2022/Non-linear 6 DOF model/MATLAB Function ==
  data: r input; y output; rot input; pod parameter
function y = pos2ag3D(r, rot, pod)
% Computes the airgaps as a function of the position and the attitude
% ═════════════════════════════════════════════════════════════════════════
% Last updated: 02.02.2022
% ═════════════════════════════════════════════════════════════════════════

y_CG  = r(1);
z_CG  = r(2);
rot_x = rot(1);
rot_y = rot(2);
rot_z = rot(3); 

AG_0  = 10e-3;

AG_1  = z_CG  -  pod.geometry.z_LEV * cos(rot_y)  -  pod.geometry.x_LEV_front * sin(rot_y)  +  pod.geometry.y_LEV * sin(rot_x);
AG_2  = z_CG  -  pod.geometry.z_LEV * cos(rot_y)                                            +  pod.geometry.y_LEV * sin(rot_x);
AG_3  = z_CG  -  pod.geometry.z_LEV * cos(rot_y)  +  pod.geometry.x_LEV_rear  * sin(rot_y)   +  pod.geometry.y_LEV * sin(rot_x);
AG_4  = z_CG  -  pod.geometry.z_LEV * cos(rot_y)  -  pod.geometry.x_LEV_front * sin(rot_y)  -  pod.geometry.y_LEV * sin(rot_x);
AG_5  = z_CG  -  pod.geometry.z_LEV * cos(rot_y)                                            -  pod.geometry.y_LEV * sin(rot_x);
AG_6  = z_CG  -  pod.geometry.z_LEV * cos(rot_y)  +  pod.geometry.x_LEV_rear  * sin(rot_y)  -  pod.geometry.y_LEV * sin(rot_x);

AG_7  = - y_CG  - pod.geometry.x_G_front * sin(rot_z) + AG_0;
AG_8  = - y_CG  + pod.geometry.x_G_rear  * sin(rot_z) + AG_0;
AG_9  =   y_CG  + pod.geometry.x_G_front * sin(rot_z) + AG_0;
AG_10 =   y_CG  - pod.geometry.x_G_rear  * sin(rot_z) + AG_0;

y = [AG_1; AG_2; AG_3; AG_4; AG_5; AG_6; AG_7; AG_8; AG_9; AG_10];

y(y<0)=0;
